simulink model "soc_range_doppler_proc"  (R2023b)
settings: Solver=FixedStepDiscrete  StartTime=0.0  StopTime=inf  RelTol=1e-3  EnableMultiTasking=on
model workspace (MAT data in the model file):
  mwTaskManagerKernelLatency = 0
values from neighbouring files (symbols this model uses):
  FPGAClkRate = Fs/SamplesPerClockCycle    (= 125000000)    [soc_range_doppler_init.m]
  TargetEmulator_InfoStruct = struct    [soc_range_doppler_init.m]
  TargetEmulator_NCO_accum_wl = 32    [soc_range_doppler_init.m]
  TargetEmulator_NumChannels = 4    [soc_range_doppler_init.m]
  TargetEmulator_NumSteps = 200    [soc_range_doppler_init.m]
  TargetEmulator_UpdateTime = 0.01    [soc_range_doppler_init.m]
  TargetInfo = TargetEmulator_InfoStruct    [soc_range_doppler_init.m]
  TsTargetUpdate = TargetEmulator_UpdateTime    (= 0.01)    [soc_range_doppler_init.m]
  udp_cmd = struct()    [soc_range_doppler_init.m]
undefined symbols (not defined in the file or in its folder): lambda, propSpeed, RngDimLen, RngMaxIdx, Ts, VelDimLen
libraries: prociolib x10, simulink x3, dspxfrm3 x1, socsharedlib_internal x1
settings Model: DataTypeOverride=Off  ModifiedByFormat=The MathWorks, Inc.  Creator=The MathWorks, Inc.  LastModifiedBy=The MathWorks, Inc.
settings SolverCC: ConcurrentTasks=on  AlgebraicLoopSolver=TrustRegion  PositivePriorityOrder=on  MaxZcPerStep=1
settings DataIOCC: LimitDataPoints=on  SaveFormat=Array  SaveOutput=off  SaveTime=off  ReturnWorkspaceOutputs=off
settings OptimizationCC: BlockReduction=off  ConditionallyExecuteInputs=off  EnhancedBackFolding=on  PassReuseOutputArgsAs=Individual arguments  ZeroExternalMemoryAtStartup=off  ZeroInternalMemoryAtStartup=off  MaxStackSize=64  OptimizeBlockOrder=speed  DifferentSizesBufferReuse=on  OptimizationCustomize=off  EfficientTunableParamExpr=on
settings DebuggingCC: AlgebraicLoopMsg=error  SolverPrmCheckMsg=warning  InheritedTsInSrcMsg=none  SingleTaskRateTransMsg=error  IntegerOverflowMsg=none  ParameterPrecisionLossMsg=none  ParameterTunabilityLossMsg=error  UnconnectedInputMsg=warning  UnconnectedOutputMsg=warning  UnconnectedLineMsg=warning  AllowSymbolicDim=off  SFUnexpectedBacktrackingDiag=warning  SFNoUnconditionalDefaultTransitionDiag=warning  SFExecutionAtInitializationDiag=none  IntegerSaturationMsg=none  ArithmeticOperatorsInVariantConditions=warning
settings HardwareCC: ProdBitPerLong=64  ProdLargestAtomicInteger=LongLong  ProdLargestAtomicFloat=Double  ProdLongLongMode=on  ProdHWDeviceType=ARM Compatible->ARM 64-bit (LP64)  TargetBitPerLong=64  TargetBitPerPointer=64  TargetBitPerSizeT=64  TargetBitPerPtrDiffT=64  TargetLargestAtomicInteger=LongLong  TargetLargestAtomicFloat=Double  TargetLongLongMode=on  TargetIntDivRoundTo=Zero  TargetEndianess=LittleEndian  TargetWordSize=64  TargetHWDeviceType=ARM Compatible->ARM 64-bit (LP64)  ProdEqTarget=off  HardwareBoardFeatureSet=SoCBlockset
settings ModelReferenceCC: EnableRefExpFcnMdlSchedulingChecks=on  ModelReferenceNumInstancesAllowed=Single  PropagateSignalLabelsOutOfModel=off
settings SFSimCC: SimUseLocalCustomCode=off  MATLABDynamicMemAlloc=off  CustomCodeUndefinedFunction=UseInterfaceOnly
settings RTWCC: Description=Embedded Coder  SystemTargetFile=ert.tlc  HardwareBoard=Xilinx Zynq UltraScale+ RFSoC ZCU111 Evaluation Kit  TLCOptions="-aInlineSetEventsForThisBaseRateFcn=TLC_FALSE -aSuppressMultiTaskScheduler=TLC_FALSE  -aRateBasedStepFcn=0"  TemplateMakefile=ert_default_tmf  RTWUseLocalCustomCode=off  Toolchain=Linaro AArch64 Linux v6.3.1  DLArmComputeVersion=19.05
settings CodeAppCC: ForceParamTrailComments=on  IgnoreCustomStorageClasses=off  OperatorAnnotations=on  SimulinkDataObjDesc=on  SFDataObjDesc=on  InsertBlockDesc=on
settings ERTTargetCC: SupportVariableSizeSignals=on
settings ConfigComp: CovMetricSettings=dw  CovSaveCumulativeToWorkspaceVar=on  CovSaveSingleToWorkspaceVar=on  CovExternalEMLEnable=off  CovSFcnEnable=off
settings SimscapeCC: SimscapeNormalizeSystem=off

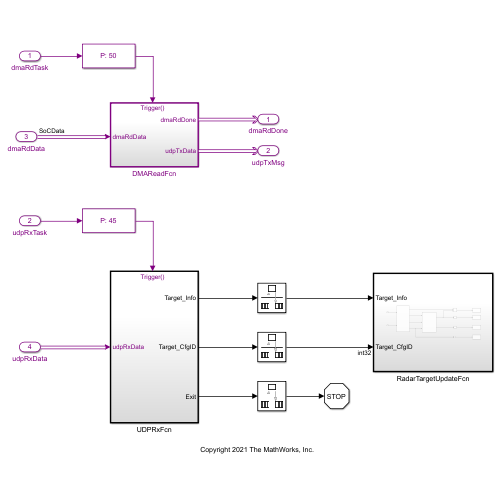
[thumbnail: Simulink's stored preview of the top-level diagram]
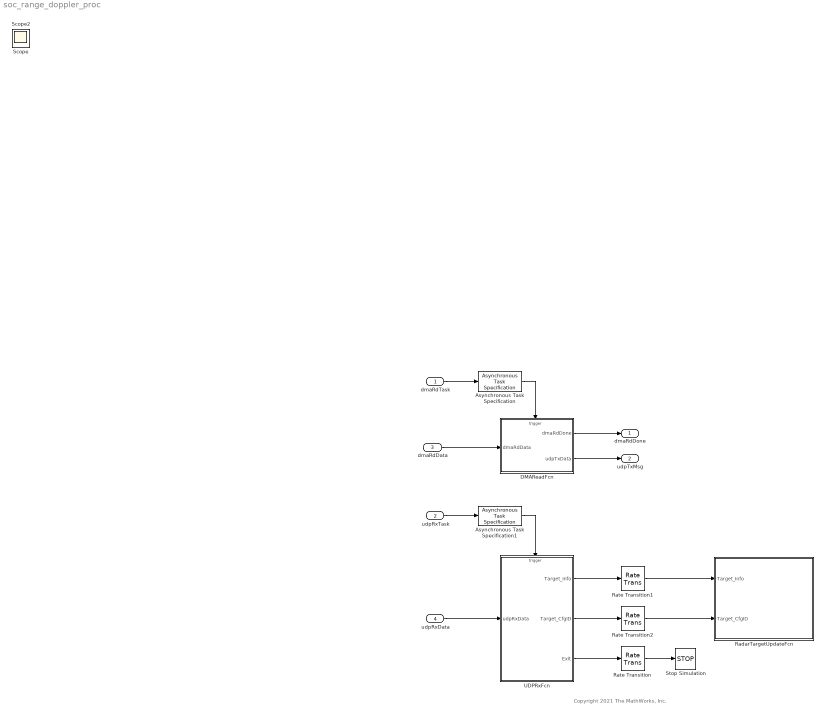
== system soc_range_doppler_proc ==
  note: Copyright 2021 The MathWorks, Inc.
  dmaRdTask : Inport  OutputFunctionCall=on
  udpRxTask : Inport  Port=2  OutputFunctionCall=on
  dmaRdData : Inport  OutputPortMessageModes=m  Port=3  OutDataTypeStr=SoCData  BusOutputAsStruct=on
  udpRxData : Inport  OutputPortMessageModes=m  Port=4
  Asynchronous Task Specification : AsynchronousTaskSpecification  TaskPriority=50
  Asynchronous Task Specification1 : AsynchronousTaskSpecification  TaskPriority=45
  DMAReadFcn : Subsystem  TreatAsAtomicUnit=on
  RadarTargetUpdateFcn : Subsystem  TreatAsAtomicUnit=on  SystemSampleTime=TsTargetUpdate
  Rate Transition : RateTransition  Deterministic=off  OutPortSampleTime=TsSWBase
  Rate Transition1 : RateTransition  Deterministic=off  OutPortSampleTime=TsTargetUpdate
  Rate Transition2 : RateTransition  Deterministic=off  OutPortSampleTime=TsTargetUpdate
  Stop Simulation : Stop
  UDPRxFcn : Subsystem  TreatAsAtomicUnit=on
  dmaRdDone : Outport  InputPortMessageModes=m  VectorParamsAs1DForOutWhenUnconnected=off
  udpTxMsg : Outport  InputPortMessageModes=m  Port=2
  Scope : Scope
  Scope2 : Scope
  wires:
  Asynchronous Task Specification/1 -> DMAReadFcn/Trigger
  dmaRdTask/1 -> Asynchronous Task Specification/1
  dmaRdData/1 -> DMAReadFcn/1(dmaRdData)
  DMAReadFcn/1(dmaRdDone) -> dmaRdDone/1
  udpRxTask/1 -> Asynchronous Task Specification1/1
  Asynchronous Task Specification1/1 -> UDPRxFcn/Trigger
  udpRxData/1 -> UDPRxFcn/1(udpRxData)
  DMAReadFcn/2(udpTxData) -> udpTxMsg/1
  Rate Transition/1 -> Stop Simulation/1
  Rate Transition1/1 -> RadarTargetUpdateFcn/1(Target_Info)
  UDPRxFcn/1(Target_Info) -> Rate Transition1/1
  UDPRxFcn/3(Exit) -> Rate Transition/1
  Rate Transition2/1 -> RadarTargetUpdateFcn/2(Target_CfgID)
  UDPRxFcn/2(Target_CfgID) -> Rate Transition2/1

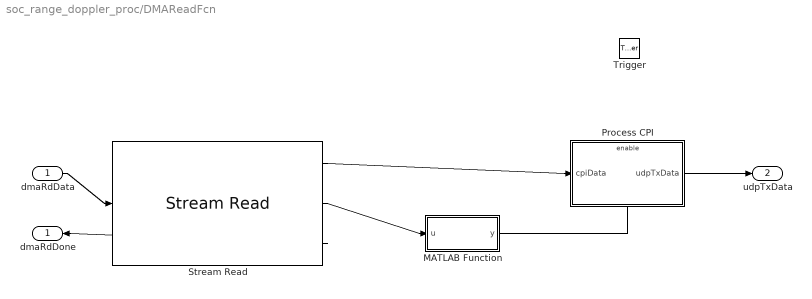
== system soc_range_doppler_proc/DMAReadFcn ==
  dmaRdData : Inport
  Trigger : TriggerPort  TriggerType=function-call  VariantControl=Variant  PortDimensions=1
  MATLAB Function : MATLAB Function  TreatAsAtomicUnit=on
  Process CPI : Subsystem  TreatAsAtomicUnit=on
  Stream Read : prociolib/Stream Read  Priority=1  DeviceName=mwrange_doppler_tx_rx_ip0:s2mm0  OutDataTypeStr=uint64  SamplesPerFrame=S2MM_DMAFrameLength  NumberOfBuffers=S2MM_DMANumBuffers  EnableEvent=on  SampleTime=-1
  dmaRdDone : Outport  VectorParamsAs1DForOutWhenUnconnected=off
  udpTxData : Outport  Port=2
  wires:
  dmaRdData/1 -> Stream Read/1
  Stream Read/3 -> dmaRdDone/1
  Stream Read/2 -> MATLAB Function/1(u)
  Process CPI/1(udpTxData) -> udpTxData/1
  Stream Read/1 -> Process CPI/1(cpiData)
  MATLAB Function/1(y) -> Process CPI/Enable

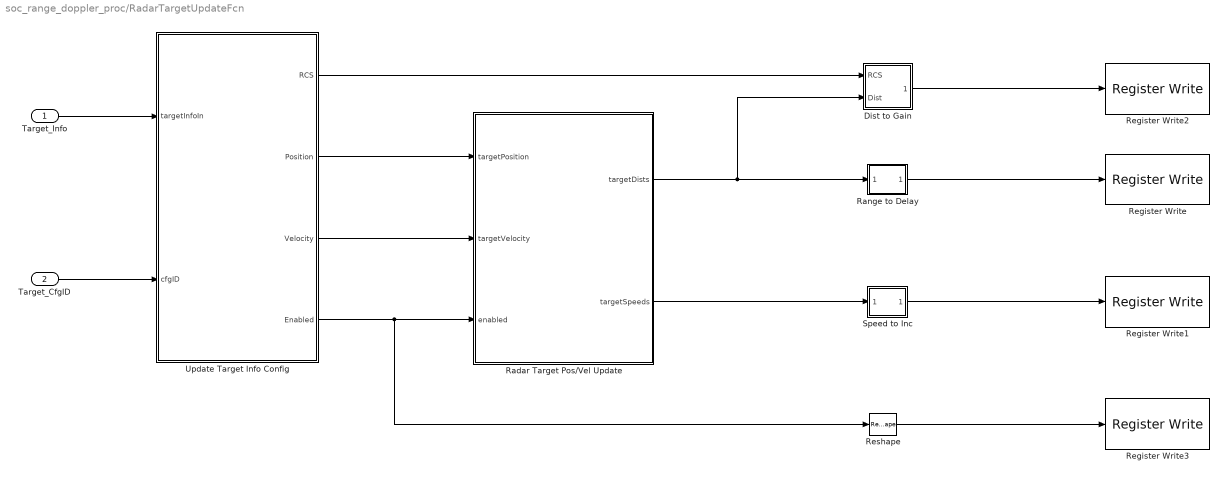
== system soc_range_doppler_proc/RadarTargetUpdateFcn ==
  Target_Info : Inport  OutDataTypeStr=Bus: TargetEmulatorInfo
  Target_CfgID : Inport  Port=2  OutDataTypeStr=int32
  Dist to Gain : Subsystem
  Radar Target Pos/Vel Update : MATLAB Function  TreatAsAtomicUnit=on  mask{timeIntvl=TargetEmulator_UpdateTime, numSteps=TargetEmulator_NumSteps, numTargets=TargetEmulator_NumChannels}
      mask prompts: timeIntvl "Time interval:"; numSteps "Number of steps:"; numTargets "Max number of target:"
  Range to Delay : Subsystem
  Register Write : prociolib/Register Write  OutputSink=IP core register  TunableParamName=A  RegisterName=Target_Emulator_Range_Delay  DeviceName=/dev/mwradar_target_emulator_ip0  OffsetAddress=hex2dec('0120')  Dummy=0
  Register Write1 : prociolib/Register Write  OutputSink=IP core register  TunableParamName=A  RegisterName=Target_Emulator_Doppler_Inc  DeviceName=/dev/mwradar_target_emulator_ip0  OffsetAddress=hex2dec('0100')  Dummy=0
  Register Write2 : prociolib/Register Write  OutputSink=IP core register  TunableParamName=A  RegisterName=Target_Emulator_Gain  DeviceName=/dev/mwradar_target_emulator_ip0  OffsetAddress=hex2dec('0140')  Dummy=0
  Register Write3 : prociolib/Register Write  OutputSink=IP core register  TunableParamName=A  RegisterName=Target_Emulator_Channel_Enable  DeviceName=/dev/mwradar_target_emulator_ip0  OffsetAddress=hex2dec('0160')  Dummy=0
  Reshape : Reshape
  Speed to Inc : Subsystem
  Update Target Info Config : MATLAB Function  TreatAsAtomicUnit=on  mask{targetInfoInit=TargetInfo}
      mask prompts: targetInfoInit "Initial config:"
  wires:
  Radar Target Pos/Vel Update/1(targetDists) -> Range to Delay/1(In1), Dist to Gain/2(Dist)
  Radar Target Pos/Vel Update/2(targetSpeeds) -> Speed to Inc/1(In1)
  Speed to Inc/1(Out1) -> Register Write1/1
  Range to Delay/1(Out1) -> Register Write/1
  Dist to Gain/1(Out1) -> Register Write2/1
  Reshape/1 -> Register Write3/1
  Target_Info/1 -> Update Target Info Config/1(targetInfoIn)
  Target_CfgID/1 -> Update Target Info Config/2(cfgID)
  Update Target Info Config/1(RCS) -> Dist to Gain/1(RCS)
  Update Target Info Config/4(Enabled) -> Radar Target Pos/Vel Update/3(enabled), Reshape/1
  Update Target Info Config/2(Position) -> Radar Target Pos/Vel Update/1(targetPosition)
  Update Target Info Config/3(Velocity) -> Radar Target Pos/Vel Update/2(targetVelocity)

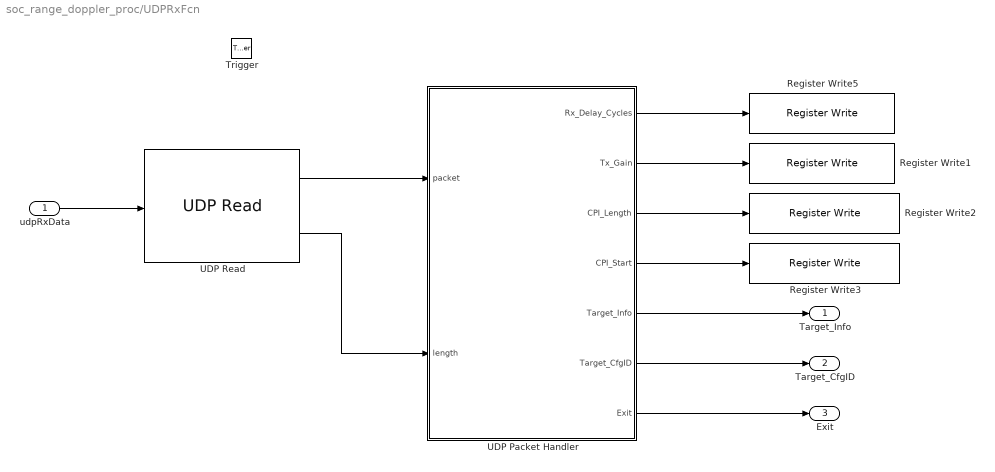
== system soc_range_doppler_proc/UDPRxFcn ==
  udpRxData : Inport
  Trigger : TriggerPort  TriggerType=function-call  VariantControl=Variant  PortDimensions=1
  Register Write1 : prociolib/Register Write  OutputSink=IP core register  TunableParamName=A  RegisterName=Tx_Gain  DeviceName=/dev/mwrange_doppler_tx_rx_ip0  OffsetAddress=hex2dec('0100')  Dummy=0
  Register Write2 : prociolib/Register Write  OutputSink=IP core register  TunableParamName=A  RegisterName=CPI_Length  DeviceName=/dev/mwrange_doppler_tx_rx_ip0  OffsetAddress=hex2dec('0108')  Dummy=0
  Register Write3 : prociolib/Register Write  OutputSink=IP core register  TunableParamName=A  RegisterName=CPI_Start  DeviceName=/dev/mwrange_doppler_tx_rx_ip0  OffsetAddress=hex2dec('0104')  Dummy=0
  Register Write5 : prociolib/Register Write  OutputSink=IP core register  TunableParamName=A  RegisterName=Rx_Delay_Cycles  DeviceName=/dev/mwrange_doppler_tx_rx_ip0  OffsetAddress=hex2dec('010C')  Dummy=0
  UDP Packet Handler : MATLAB Function  TreatAsAtomicUnit=on
  UDP Read : prociolib/UDP Read  LocalPort=25001  DataType=double  DataLength=udp_cmd.MessageLength  ReceiveBufferSize=65535  ByteOrder=LittleEndian  EnableEvent=on  OutputVarSizeSignal=off  OutputStatus=off  SampleTime=-1  hoistedMaskSrc=Variant/CODEGEN/UDP Read
  Target_Info : Outport
  Target_CfgID : Outport  Port=2  InitialOutput=0
  Exit : Outport  Port=3
  wires:
  UDP Read/2 -> UDP Packet Handler/2(length)
  udpRxData/1 -> UDP Read/1
  UDP Read/1 -> UDP Packet Handler/1(packet)
  UDP Packet Handler/4(CPI_Start) -> Register Write3/1
  UDP Packet Handler/3(CPI_Length) -> Register Write2/1
  UDP Packet Handler/2(Tx_Gain) -> Register Write1/1
  UDP Packet Handler/7(Exit) -> Exit/1
  UDP Packet Handler/1(Rx_Delay_Cycles) -> Register Write5/1
  UDP Packet Handler/5(Target_Info) -> Target_Info/1
  UDP Packet Handler/6(Target_CfgID) -> Target_CfgID/1

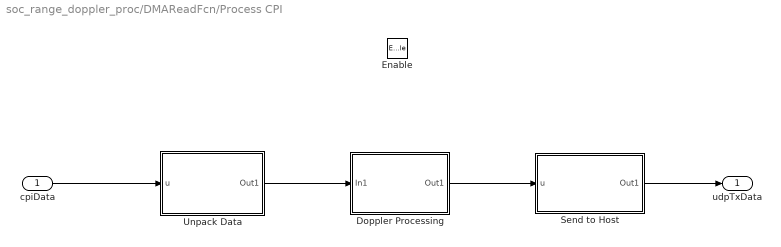
== system soc_range_doppler_proc/DMAReadFcn/Process CPI ==
  cpiData : Inport
  Enable : EnablePort
  Doppler Processing : Subsystem  TreatAsAtomicUnit=on
  Send to Host : Subsystem  TreatAsAtomicUnit=on
  Unpack Data : Subsystem  TreatAsAtomicUnit=on
  udpTxData : Outport
  wires:
  cpiData/1 -> Unpack Data/1(u)
  Unpack Data/1(Out1) -> Doppler Processing/1(In1)
  Doppler Processing/1(Out1) -> Send to Host/1(u)
  Send to Host/1(Out1) -> udpTxData/1

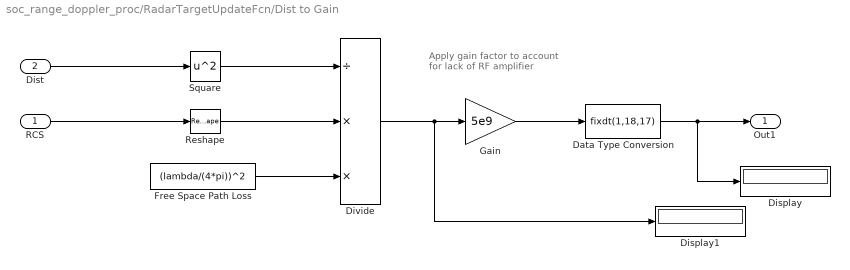
== system soc_range_doppler_proc/RadarTargetUpdateFcn/Dist to Gain ==
  note: Apply gain factor to account
      | for lack of RF amplifier
  RCS : Inport
  Dist : Inport  Port=2
  Data Type Conversion : DataTypeConversion  OutDataTypeStr=fixdt(1,18,17)  SaturateOnIntegerOverflow=off  RndMeth=Floor
  Display : Display
  Display1 : Display
  Divide : Product  Inputs=/**  RndMeth=Zero  SaturateOnIntegerOverflow=on
  Free Space Path Loss : Constant  Value=(lambda/(4*pi))^2  OutDataTypeStr=single  SampleTime=-1
  Gain : Gain  Gain=5e9
  Reshape : Reshape
  Square : Math  Operator=square
  Out1 : Outport
  wires:
  Data Type Conversion/1 -> Out1/1, Display/1
  Dist/1 -> Square/1
  Square/1 -> Divide/1
  Free Space Path Loss/1 -> Divide/3
  Divide/1 -> Display1/1, Gain/1
  Gain/1 -> Data Type Conversion/1
  RCS/1 -> Reshape/1
  Reshape/1 -> Divide/2

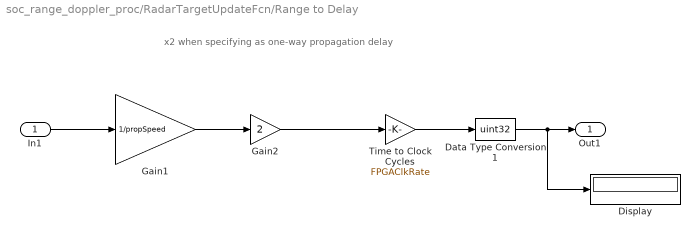
== system soc_range_doppler_proc/RadarTargetUpdateFcn/Range to Delay ==
  note: x2 when specifying as one-way propagation delay
  In1 : Inport
  Data Type Conversion1 : DataTypeConversion  OutDataTypeStr=uint32  SaturateOnIntegerOverflow=off  RndMeth=Floor
  Display : Display
  Gain1 : Gain  Gain=1/propSpeed
  Gain2 : Gain  Gain=2
  Time to Clock Cycles : Gain  Gain=FPGAClkRate
  Out1 : Outport
  wires:
  Data Type Conversion1/1 -> Display/1, Out1/1
  Time to Clock Cycles/1 -> Data Type Conversion1/1
  In1/1 -> Gain1/1
  Gain1/1 -> Gain2/1
  Gain2/1 -> Time to Clock Cycles/1

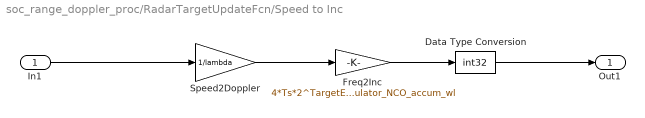
== system soc_range_doppler_proc/RadarTargetUpdateFcn/Speed to Inc ==
  In1 : Inport
  Data Type Conversion : DataTypeConversion  OutDataTypeStr=int32  SaturateOnIntegerOverflow=off  RndMeth=Floor
  Freq2Inc : Gain  Gain=4*Ts*2^TargetEmulator_NCO_accum_wl
  Speed2Doppler : Gain  Gain=1/lambda
  Out1 : Outport
  wires:
  Freq2Inc/1 -> Data Type Conversion/1
  Speed2Doppler/1 -> Freq2Inc/1
  Data Type Conversion/1 -> Out1/1
  In1/1 -> Speed2Doppler/1

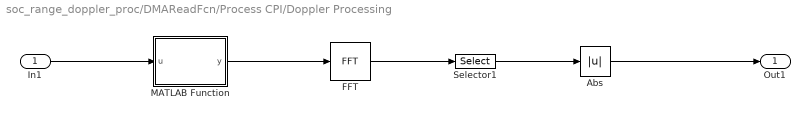
== system soc_range_doppler_proc/DMAReadFcn/Process CPI/Doppler Processing ==
  In1 : Inport
  Abs : Abs  SaturateOnIntegerOverflow=off
  FFT : dspxfrm3/FFT  FFTImplementation=Auto  CompMethod=Table lookup  TableOpt=NEW  TableOptActive=Speed  BitRevOrder=off  Normalize=off  InheritFFTLength=on  FFTLength=64  WrapInput=on  roundingMode=Floor  overflowMode=off  firstCoeffDataTypeStr=Inherit: Same word length as input  firstCoeffLastDataTypeStr=Inherit: Same word length as input  outputMin=[]  outputMax=[]
  MATLAB Function : MATLAB Function  TreatAsAtomicUnit=on
  Selector1 : Selector  NumberOfDimensions=2  InputPortWidth=3  IndexOptions=Select all,Index vector (dialog)  Indices=[1:RngMaxIdx],[1:RngMaxIdx]  OutputSizes=1,1
  Out1 : Outport
  wires:
  FFT/1 -> Selector1/1
  In1/1 -> MATLAB Function/1(u)
  Abs/1 -> Out1/1
  MATLAB Function/1(y) -> FFT/1
  Selector1/1 -> Abs/1

== system soc_range_doppler_proc/DMAReadFcn/Process CPI/Send to Host ==
  u : Inport
  UDP Write : Subsystem  mask(UDP Write){RemoteAddress=255.255.255.255, RemotePort=25000, LocalPort=-1, ByteOrder=LittleEndian, OutputStatus=off, hoistedMaskSrc=Variant/CODEGEN/For Loop/UDP Write}
      mask prompts: RemoteAddress "Remote IP address (255.255.255.255 for broadcast):"; RemotePort "Remote IP port:"; LocalPort "Local IP port:"; ByteOrder "Byte order:"; OutputStatus "Enable status output port"
      mask help:
      | Send UDP packets to a specified remote IP address and port.
      |
      | The block accepts a one-dimensional array of type uint8, int8, uint16, int16, uint32, int32, single, or double.
      |
      | Set the Remote IP address and Remote IP port parameters to the IP address and port of the host where UDP data is to be sent. Set the Local IP port to -1 to use a random available port number to send packets.
      mask init:
      | soc.internal.UDPWriteCb('MaskInitFcn',gcbh');
      mask Help: eval('soc.internal.helpview(''soc_udpwrite'')')
      mask TypeOptions RemoteAddress: Variant/CODEGEN/For Loop/UDP Write/RemoteAddress
      mask TypeOptions RemotePort: Variant/CODEGEN/For Loop/UDP Write/RemotePort
      mask TypeOptions LocalPort: Variant/CODEGEN/For Loop/UDP Write/LocalPort
      mask TypeOptions ByteOrder: Variant/CODEGEN/For Loop/UDP Write/ByteOrder
      mask TypeOptions OutputStatus: Variant/CODEGEN/For Loop/UDP Write/OutputStatus
      mask DialogControl Container9 Prompt: Parameters
      mask Display:
      | color('white');
      | plot([100,100,100,100],[100,100,100,100]);
      | plot([0,0,0,0],[0,0,0,0]);
      | color('blue');
      | text(99, 92, '', 'horizontalAlignment', 'right');
      | color('black');
      | text(50, 30, [sprintf('Addr: %s','255.255.255.255')],'texmode','off','horizontalAlignment','center','verticalAlignment','middle');
      | text(50, 15,[sprintf('Port: %s','25000')],'texmode','off','horizontalAlignment','center','verticalAlignment','middle');
      | port_label('input',1,'');
      | 
      | 
      | port_label('input', 1, 'data')
      | port_label('output', 1, 'msg')
  Out1 : Outport
  wires:
  UDP Write/1(Message) -> Out1/1
  u/1 -> UDP Write/1(Data)

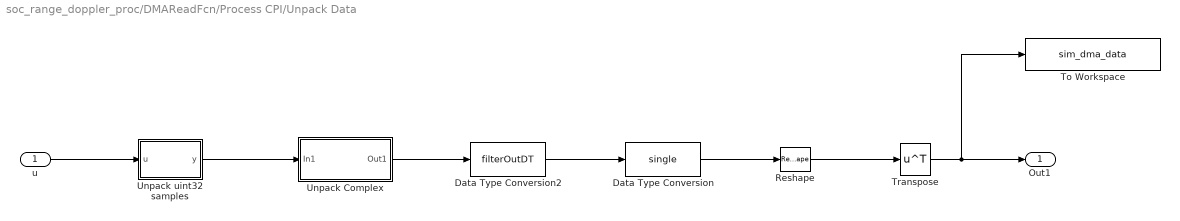
== system soc_range_doppler_proc/DMAReadFcn/Process CPI/Unpack Data ==
  u : Inport
  Data Type Conversion : DataTypeConversion  OutDataTypeStr=single  SaturateOnIntegerOverflow=off  RndMeth=Floor
  Data Type Conversion2 : DataTypeConversion  OutDataTypeStr=filterOutDT  ConvertRealWorld=Stored Integer (SI)  SaturateOnIntegerOverflow=off  RndMeth=Floor
  Reshape : Reshape  OutputDimensionality=Customize  OutputDimensions=[RngDimLen VelDimLen]
  To Workspace : ToWorkspace  VariableName=sim_dma_data  SampleTime=-1
  Transpose : Math  Operator=transpose
  Unpack Complex : Subsystem
  Unpack uint32 samples : MATLAB Function  TreatAsAtomicUnit=on
  Out1 : Outport
  wires:
  Data Type Conversion2/1 -> Data Type Conversion/1
  Unpack Complex/1(Out1) -> Data Type Conversion2/1
  Reshape/1 -> Transpose/1
  Unpack uint32 samples/1(y) -> Unpack Complex/1(In1)
  u/1 -> Unpack uint32 samples/1(u)
  Data Type Conversion/1 -> Reshape/1
  Transpose/1 -> To Workspace/1, Out1/1

== system soc_range_doppler_proc/DMAReadFcn/Process CPI/Send to Host/UDP Write ==
  Data : Inport
  Variant : Subsystem  Tag=_uses_sim_codegen_variant_  Variant=on  VariantControlMode=sim codegen switching
  Message : Outport  VectorParamsAs1DForOutWhenUnconnected=off
  wires:
  Variant/1(Message) -> Message/1
  Data/1 -> Variant/1("Data ")

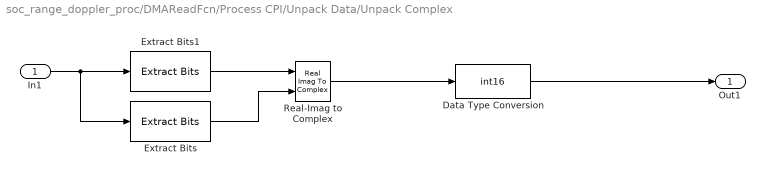
== system soc_range_doppler_proc/DMAReadFcn/Process CPI/Unpack Data/Unpack Complex ==
  In1 : Inport
  Data Type Conversion : DataTypeConversion  OutDataTypeStr=int16  ConvertRealWorld=Stored Integer (SI)  SaturateOnIntegerOverflow=off  RndMeth=Floor
  Extract Bits : simulink/Logic and Bit Operations/Extract Bits  bitsToExtract=Upper half  numBits=8  bitIdxRange=[0 7]  outScalingMode=Treat bit field as an integer
  Extract Bits1 : simulink/Logic and Bit Operations/Extract Bits  bitsToExtract=Lower half  numBits=8  bitIdxRange=[0 7]  outScalingMode=Treat bit field as an integer
  Real-Imag to Complex : RealImagToComplex
  Out1 : Outport
  wires:
  In1/1 -> Extract Bits/1, Extract Bits1/1
  Extract Bits1/1 -> Real-Imag to Complex/1
  Real-Imag to Complex/1 -> Data Type Conversion/1
  Extract Bits/1 -> Real-Imag to Complex/2
  Data Type Conversion/1 -> Out1/1

== system soc_range_doppler_proc/DMAReadFcn/Process CPI/Send to Host/UDP Write/Variant ==
  "Data " : Inport
  CODEGEN : Subsystem  VariantControl=(codegen)
  SIM : Subsystem  VariantControl=(sim)
  Message : Outport  VectorParamsAs1DForOutWhenUnconnected=off

== system soc_range_doppler_proc/DMAReadFcn/Process CPI/Send to Host/UDP Write/Variant/CODEGEN ==
  Data : Inport
  For Loop : Subsystem  TreatAsAtomicUnit=on
  wires:
  Data/1 -> For Loop/1(In1)

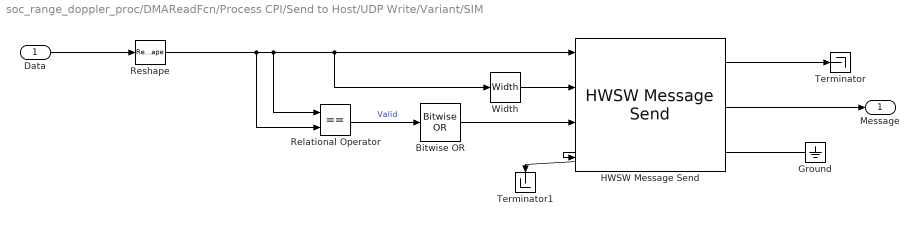
== system soc_range_doppler_proc/DMAReadFcn/Process CPI/Send to Host/UDP Write/Variant/SIM ==
  "Data " : Inport
  Bitwise OR : simulink/Logic and Bit Operations/Bitwise Operator  logicop=OR  UseBitMask=off  BitMask=bin2dec('11011001')  BitMaskRealWorld=Stored Integer
  Ground : Ground
  HWSW Message Send : socsharedlib_internal/HWSW Message Send  QueueLength=1  MessageType=UDP  MessageID=HWSWMetadataID.UDP  EnableEventPort=off  EnableDonePort=off
  Relational Operator : RelationalOperator  Operator===  OutDataTypeStr=boolean  RndMeth=Simplest  InputSameDT=off
  Reshape : Reshape
  Terminator : Terminator
  Terminator1 : Terminator
  Width : Width  DataType=uint32
  Message : Outport  VectorParamsAs1DForOutWhenUnconnected=off
  wires:
  Ground/1 -> HWSW Message Send/4
  HWSW Message Send/3 -> Terminator1/1
  HWSW Message Send/1 -> Terminator/1
  HWSW Message Send/2 -> Message/1
  Width/1 -> HWSW Message Send/2
  Bitwise OR/1 -> HWSW Message Send/3
  Relational Operator/1 -> Bitwise OR/1  "Valid"
  Reshape/1 -> HWSW Message Send/1, Width/1, Relational Operator/1, Relational Operator/2
  "Data "/1 -> Reshape/1

== system soc_range_doppler_proc/DMAReadFcn/Process CPI/Send to Host/UDP Write/Variant/CODEGEN/For Loop ==
  In1 : Inport
  For Iterator : ForIterator  IterationLimit=VelDimLen
  MATLAB Function : MATLAB Function  TreatAsAtomicUnit=on
  Selector : Selector  NumberOfDimensions=2  InputPortWidth=3  IndexOptions=Index vector (port),Select all  Indices=[1 3],1  OutputSizes=1,1
  UDP Write : MATLABSystem  System=soc.linux.UDPWrite  RemoteAddress=255.255.255.255  RemotePort=RemotePort  LocalPort=LocalPort  SendBufferSize=-1  ByteOrder=LittleEndian  OutputStatus=off  SendSimulationInputTo=Terminator
      mask Type: soc.linux.UDPWrite
      mask Display:
      | color('white');
      | plot([100,100,100,100],[100,100,100,100]);
      | plot([0,0,0,0],[0,0,0,0]);
      | color('blue');
      | text(99, 92, '', 'horizontalAlignment', 'right');
      | color('black');
      | text(50, 30, [sprintf('Addr: %s','255.255.255.255')],'texmode','off','horizontalAlignment','center','verticalAlignment','middle');
      | text(50, 15,[sprintf('Port: %s','25000')],'texmode','off','horizontalAlignment','center','verticalAlignment','middle');
      | port_label('input',1,'');
  wires:
  Selector/1 -> UDP Write/1
  In1/1 -> Selector/1
  For Iterator/1 -> MATLAB Function/1(idx), Selector/2

== matlab function soc_range_doppler_proc/UDPRxFcn/UDP Packet Handler ==
  data: Rx_Delay_Cycles output; Tx_Gain output; CPI_Length output; CPI_Start output; Target_Info output Bus: TargetEmulatorInfo; Target_CfgID output; Exit output; packet input; length input; udp_cmd parameter; TargetEmulator_InfoStruct parameter; TargetEmulator_NumChannels parameter
function [Rx_Delay_Cycles, Tx_Gain, CPI_Length, CPI_Start, Target_Info, Target_CfgID, Exit]= ...
    handle_udp_packet(packet, length, udp_cmd, TargetEmulator_InfoStruct, TargetEmulator_NumChannels)

persistent Rx_Delay_Cycles_p Tx_Gain_p CPI_Length_p Exit_p Target_Info_p Target_CfgID_p
if isempty(Tx_Gain_p)
    Rx_Delay_Cycles_p = uint32(0);
    Tx_Gain_p = fi(0, 1,18,16);
    CPI_Length_p = uint32(0);
    Exit_p = false;
    Target_Info_p = TargetEmulator_InfoStruct;
    Target_CfgID_p = int32(0);
end

cmd = packet(1);
data = packet(2:end);

% default value
CPI_Start = false;

if (length == udp_cmd.MessageLength)
    switch cmd
        case udp_cmd.Rx_Delay_Cycles
            l_print('Setting Rx delay cycles to %d',int32(data(1)));
            Rx_Delay_Cycles_p(:) = data(1);
        case udp_cmd.Tx_Gain
            l_print('Setting Tx gain to %.3f',data(1));
            Tx_Gain_p(:) = data(1);
        case udp_cmd.CPI_Length
            l_print('Setting CPI length to %d',int32(data(1)));
            CPI_Length_p(:) = data(1)-1;
        case udp_cmd.CPI_Start
            if data(1)
                l_print('Starting CPI...');
            end
            CPI_Start(:) = data(1);
        case udp_cmd.Target_Info
            idx = data(1);
            if (idx > 0) && (idx <= TargetEmulator_NumChannels)
                l_print('Configuring radar target channel %d',int32(idx));
                Target_Info_p.Enabled(idx) = data(2);
                Target_Info_p.Position(:,idx) = data(3:5);
                Target_Info_p.Velocity(:,idx) = data(6:8);
                Target_Info_p.RCS(idx) = data(9);
            end
            Target_CfgID_p = Target_CfgID_p+1;
        case udp_cmd.Exit
            l_print('Exiting...');
            Exit_p = true;
    end
end

Rx_Delay_Cycles = Rx_Delay_Cycles_p;
Tx_Gain = Tx_Gain_p;
CPI_Length = CPI_Length_p;
Exit = Exit_p;
Target_Info = Target_Info_p;
Target_CfgID = Target_CfgID_p;

end

function l_print(str,val,nl)
    if nargin < 2
        val = [];
    end
    if nargin < 3
        nl = true;
    end
    if nl
        nlchar = newline;
    else
        nlchar = '';
    end
    if coder.target('rtw')
        if isempty(val)
            coder.ceval('printf',[str nlchar uint8(0)]);
        else
            coder.ceval('printf',[str nlchar uint8(0)],val);
        end
    else
        if isempty(val)
            fprintf([str nlchar]);
        else
            fprintf([str nlchar],val);
        end
    end
end

== matlab function soc_range_doppler_proc/DMAReadFcn/MATLAB Function ==
  data: u input; y output
function y = print_dma_valid(u)

if u
    l_print('DMA packet read');
end

y = u;

end

function l_print(str)
    if coder.target('rtw')
        coder.ceval('printf',[str uint8(10) uint8(0)]);
    else
        fprintf([str newline]);
    end
end

== matlab function soc_range_doppler_proc/DMAReadFcn/Process CPI/Send to Host/UDP Write/Variant/CODEGEN/For Loop/MATLAB Function ==
  data: idx input
function udp_status(idx)

if (idx == 1) 
    if coder.target('rtw')
        coder.ceval('printf',['Send results to host' uint8(10) uint8(0)]);
    end
end

== matlab function soc_range_doppler_proc/RadarTargetUpdateFcn/Update Target Info Config ==
  data: RCS output single; Position output single; Velocity output single; targetInfoIn input Bus: TargetEmulatorInfo; Enabled output boolean; cfgID input; targetInfoInit parameter Bus: TargetEmulatorInfo
function [RCS,Position,Velocity,Enabled] = updateTargetInfoConfig(targetInfoIn, cfgID, targetInfoInit)

persistent cfgID_p targetInfo
if isempty(cfgID_p)
    cfgID_p = int32(0);
    targetInfo = targetInfoInit;
end

% Update the target info only when we have a new config ID
if cfgID > cfgID_p
    cfgID_p = cfgID;
    targetInfo = targetInfoIn;
end

RCS = targetInfo.RCS;
Position = targetInfo.Position;
Velocity = targetInfo.Velocity;
Enabled = targetInfo.Enabled;

== matlab function soc_range_doppler_proc/DMAReadFcn/Process CPI/Doppler Processing/MATLAB Function ==
  data: u input; y output
function y = disp_proc_start(u)

if coder.target('rtw')
   coder.ceval('printf',['Begin Doppler processing' uint8(10) uint8(0)]);
end

y = u;

== matlab function soc_range_doppler_proc/RadarTargetUpdateFcn/Radar Target Pos//Vel Update ==
  data: targetPosition input; targetVelocity input; enabled input; targetDists output; targetSpeeds output; timeIntvl parameter single; numSteps parameter int32; numTargets parameter
function [targetDists, targetSpeeds] = updateTargets(targetPosition, targetVelocity, enabled, ...
    timeIntvl, numSteps, numTargets)
%# codegen

%% setup

persistent targetPosition_p targetVelocity_p enabled_p stepCount

if isempty(targetPosition_p)
    targetPosition_p    = targetPosition;
    targetVelocity_p    = targetVelocity;
    enabled_p           = enabled;
    stepCount           = int32(1);
end

targetDists     = zeros(numTargets,1,'single');
targetSpeeds    = zeros(numTargets,1,'single');

for k = 1:numTargets
    if enabled_p(k)
        % Calculate target radial velocities and distances
        [targetDists(k), targetSpeeds(k)] = ...
            to_radial(targetPosition_p(:,k), targetVelocity_p(:,k));

        % Update target position
        targetPosition_p(:,k) = targetPosition_p(:,k) + targetVelocity_p(:,k)*timeIntvl;
    end
end

% Update step count
if stepCount == numSteps
    targetPosition_p    = targetPosition;
    targetVelocity_p    = targetVelocity;
    enabled_p           = enabled;
    stepCount(:)        = 1;
else
    stepCount = stepCount+1;
end

end

function [rdist,rspeed] = to_radial(tgtpos, tgtvel)

    rdist = sqrt(sum(tgtpos.^2));
    sn = sqrt(sum(tgtvel.^2));

    % negative sign to ensure that incoming relative speed is positive
    rspeed = -(sum(tgtvel.*tgtpos)./rdist);

    %now take care of rspeed corner cases:
    rspeed(sn==0) = 0;
    % when co-located, the radial speed is relative speed, but departing
    rnEq0 = (rdist==0);
    rspeed(rnEq0) = -sn(rnEq0); 

    %make a column vector
    rspeed = reshape(rspeed, [],1); 
end

== matlab function soc_range_doppler_proc/DMAReadFcn/Process CPI/Unpack Data/Unpack uint32 samples ==
  data: u input; y output
function y = unpack_u32_samples(u)

y = typecast(u,'uint32');
